simulink model "SC_Cell_Balancing"  (R2020b)
settings: Solver=VariableStepAuto  StartTime=0.0  StopTime=3000  RelTol=1e-3
model workspace (MAT data in the model file):
  C1 = Simulink.Parameter
  C1.Value = 360
  C1.DataType = 'auto'
  C1.Dimensions = [1 1]
  C10 = Simulink.Parameter
  C10.Value = 410
  C10.DataType = 'auto'
  C10.Dimensions = [1 1]
  C11 = Simulink.Parameter
  C11.Value = 420
  C11.DataType = 'auto'
  C11.Dimensions = [1 1]
  C12 = Simulink.Parameter
  C12.Value = 432
  C12.DataType = 'auto'
  C12.Dimensions = [1 1]
  C2 = Simulink.Parameter
  C2.Value = 365
  C2.DataType = 'auto'
  C2.Dimensions = [1 1]
  C3 = Simulink.Parameter
  C3.Value = 370
  C3.DataType = 'auto'
  C3.Dimensions = [1 1]
  C4 = Simulink.Parameter
  C4.Value = 375
  C4.DataType = 'auto'
  C4.Dimensions = [1 1]
  C5 = Simulink.Parameter
  C5.Value = 380
  C5.DataType = 'auto'
  C5.Dimensions = [1 1]
  C6 = Simulink.Parameter
  C6.Value = 385
  C6.DataType = 'auto'
  C6.Dimensions = [1 1]
  C7 = Simulink.Parameter
  C7.Value = 390
  C7.DataType = 'auto'
  C7.Dimensions = [1 1]
  C8 = Simulink.Parameter
  C8.Value = 395
  C8.DataType = 'auto'
  C8.Dimensions = [1 1]
  C9 = Simulink.Parameter
  C9.Value = 400
  C9.DataType = 'auto'
  C9.Dimensions = [1 1]
  R_bal = 360
  Vsc = Simulink.Parameter
  Vsc.Value = 0
  Vsc.DataType = 'auto'
  Vsc.Dimensions = [1 1]
libraries: powerlib x36, electricdrivelib x12
settings Model: OrderedModelArguments=off  Creator=reigs  LastModifiedBy=reigs

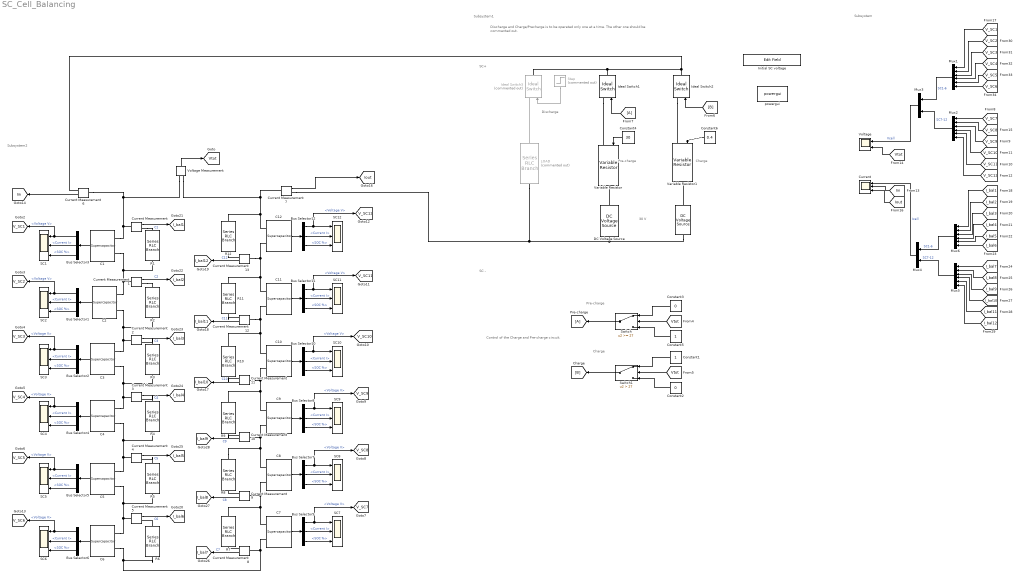
== system SC_Cell_Balancing ==
  note: Subsystem
  note: Subsystem2
  note: Subsystem1
  note: Control of the Charge and Pre-charge circuit.
  note: Charge
  note: Pre-charge
  note: SC -
  note: SC+
  note: Discharge and Charge/Precharge is to be operated only one at a time. The other one should be commented out.
  note: Discharge
  note: Pre-charge
  note: Charge
  note: 30 V
  " " : powerlib/Electrical Sources/DC Voltage Source  Amplitude=30  Measurements=None
  Bus Selector{1..12} (12 alike) : BusSelector  OutputSignals=Voltage V,Current I,SOC %
  C1 : electricdrivelib/Extra Sources/Supercapacitor  C=C1  Rdc=3.2e-3  Voltage=2.7  Ns=1  Np=1  Vinit=Vsc  Temp=25  PresetModel=off  EstParam=off  Nc=1  r=1e-9  epsilon=6.0208e-10  Ich=10  Vstern="[0.161  2.7  7.8]"  Self_dis=on  Ioc=10  Vself="[48  47.8  47.06  44.65]"  demandeplot=off  I="[10  20 100  500]"  Units=sec  Vmax=0  If=0  deltaV=0  alpha=0  sec=0
      settings: SourceProductBaseCode=PS
  C10 : electricdrivelib/Extra Sources/Supercapacitor  C=C10  Rdc=3.2e-3  Voltage=2.7  Ns=1  Np=1  Vinit=Vsc  Temp=25  PresetModel=off  EstParam=off  Nc=1  r=1e-9  epsilon=6.0208e-10  Ich=10  Vstern="[0.161  2.7  7.8]"  Self_dis=on  Ioc=10  Vself="[48  47.8  47.06  44.65]"  demandeplot=off  I="[10  20 100  500]"  Units=sec  Vmax=0  If=0  deltaV=0  alpha=0  sec=0
      settings: SourceProductBaseCode=PS
  C11 : electricdrivelib/Extra Sources/Supercapacitor  C=C11  Rdc=3.2e-3  Voltage=2.7  Ns=1  Np=1  Vinit=Vsc  Temp=25  PresetModel=off  EstParam=off  Nc=1  r=1e-9  epsilon=6.0208e-10  Ich=10  Vstern="[0.161  2.7  7.8]"  Self_dis=on  Ioc=10  Vself="[48  47.8  47.06  44.65]"  demandeplot=off  I="[10  20 100  500]"  Units=sec  Vmax=0  If=0  deltaV=0  alpha=0  sec=0
      settings: SourceProductBaseCode=PS
  C12 : electricdrivelib/Extra Sources/Supercapacitor  C=C12  Rdc=3.2e-3  Voltage=2.7  Ns=1  Np=1  Vinit=Vsc  Temp=25  PresetModel=off  EstParam=off  Nc=1  r=1e-9  epsilon=6.0208e-10  Ich=10  Vstern="[0.161  2.7  7.8]"  Self_dis=on  Ioc=10  Vself="[48  47.8  47.06  44.65]"  demandeplot=off  I="[10  20 100  500]"  Units=sec  Vmax=0  If=0  deltaV=0  alpha=0  sec=0
      settings: SourceProductBaseCode=PS
  C2 : electricdrivelib/Extra Sources/Supercapacitor  C=C2  Rdc=3.2e-3  Voltage=2.7  Ns=1  Np=1  Vinit=Vsc  Temp=25  PresetModel=off  EstParam=off  Nc=1  r=1e-9  epsilon=6.0208e-10  Ich=10  Vstern="[0.161  2.7  7.8]"  Self_dis=on  Ioc=10  Vself="[48  47.8  47.06  44.65]"  demandeplot=off  I="[10  20 100  500]"  Units=sec  Vmax=0  If=0  deltaV=0  alpha=0  sec=0
      settings: SourceProductBaseCode=PS
  C3 : electricdrivelib/Extra Sources/Supercapacitor  C=C3  Rdc=3.2e-3  Voltage=2.7  Ns=1  Np=1  Vinit=Vsc  Temp=25  PresetModel=off  EstParam=off  Nc=1  r=1e-9  epsilon=6.0208e-10  Ich=10  Vstern="[0.161  2.7  7.8]"  Self_dis=on  Ioc=10  Vself="[48  47.8  47.06  44.65]"  demandeplot=off  I="[10  20 100  500]"  Units=sec  Vmax=0  If=0  deltaV=0  alpha=0  sec=0
      settings: SourceProductBaseCode=PS
  C4 : electricdrivelib/Extra Sources/Supercapacitor  C=C4  Rdc=3.2e-3  Voltage=2.7  Ns=1  Np=1  Vinit=Vsc  Temp=25  PresetModel=off  EstParam=off  Nc=1  r=1e-9  epsilon=6.0208e-10  Ich=10  Vstern="[0.161  2.7  7.8]"  Self_dis=on  Ioc=10  Vself="[48  47.8  47.06  44.65]"  demandeplot=off  I="[10  20 100  500]"  Units=sec  Vmax=0  If=0  deltaV=0  alpha=0  sec=0
      settings: SourceProductBaseCode=PS
  C5 : electricdrivelib/Extra Sources/Supercapacitor  C=C5  Rdc=3.2e-3  Voltage=2.7  Ns=1  Np=1  Vinit=Vsc  Temp=25  PresetModel=off  EstParam=off  Nc=1  r=1e-9  epsilon=6.0208e-10  Ich=10  Vstern="[0.161  2.7  7.8]"  Self_dis=on  Ioc=10  Vself="[48  47.8  47.06  44.65]"  demandeplot=off  I="[10  20 100  500]"  Units=sec  Vmax=0  If=0  deltaV=0  alpha=0  sec=0
      settings: SourceProductBaseCode=PS
  C6 : electricdrivelib/Extra Sources/Supercapacitor  C=C6  Rdc=3.2e-3  Voltage=2.7  Ns=1  Np=1  Vinit=Vsc  Temp=25  PresetModel=off  EstParam=off  Nc=1  r=1e-9  epsilon=6.0208e-10  Ich=10  Vstern="[0.161  2.7  7.8]"  Self_dis=on  Ioc=10  Vself="[48  47.8  47.06  44.65]"  demandeplot=off  I="[10  20 100  500]"  Units=sec  Vmax=0  If=0  deltaV=0  alpha=0  sec=0
      settings: SourceProductBaseCode=PS
  C7 : electricdrivelib/Extra Sources/Supercapacitor  C=C7  Rdc=3.2e-3  Voltage=2.7  Ns=1  Np=1  Vinit=Vsc  Temp=25  PresetModel=off  EstParam=off  Nc=1  r=1e-9  epsilon=6.0208e-10  Ich=10  Vstern="[0.161  2.7  7.8]"  Self_dis=on  Ioc=10  Vself="[48  47.8  47.06  44.65]"  demandeplot=off  I="[10  20 100  500]"  Units=sec  Vmax=0  If=0  deltaV=0  alpha=0  sec=0
      settings: SourceProductBaseCode=PS
  C8 : electricdrivelib/Extra Sources/Supercapacitor  C=C8  Rdc=3.2e-3  Voltage=2.7  Ns=1  Np=1  Vinit=Vsc  Temp=25  PresetModel=off  EstParam=off  Nc=1  r=1e-9  epsilon=6.0208e-10  Ich=10  Vstern="[0.161  2.7  7.8]"  Self_dis=on  Ioc=10  Vself="[48  47.8  47.06  44.65]"  demandeplot=off  I="[10  20 100  500]"  Units=sec  Vmax=0  If=0  deltaV=0  alpha=0  sec=0
      settings: SourceProductBaseCode=PS
  C9 : electricdrivelib/Extra Sources/Supercapacitor  C=C9  Rdc=3.2e-3  Voltage=2.7  Ns=1  Np=1  Vinit=Vsc  Temp=25  PresetModel=off  EstParam=off  Nc=1  r=1e-9  epsilon=6.0208e-10  Ich=10  Vstern="[0.161  2.7  7.8]"  Self_dis=on  Ioc=10  Vself="[48  47.8  47.06  44.65]"  demandeplot=off  I="[10  20 100  500]"  Units=sec  Vmax=0  If=0  deltaV=0  alpha=0  sec=0
      settings: SourceProductBaseCode=PS
  Constant1 : Constant
  Constant2 : Constant  Value=0
  Constant3 : Constant  Value=0
  Constant4 : Constant  Value=30
  Constant5 : Constant
  Constant6 : Constant  Value=0.4
  Current : Scope  NumInputPorts=3
  Current Measurement{,1..13} (14 alike) : powerlib/Measurements/Current Measurement  PhasorSimulation=off  OutputType=Complex  PSBequivalent=0
  DC Voltage Source : powerlib/Electrical Sources/DC Voltage Source  Amplitude=30  Measurements=None
  Ideal Switch1 : powerlib/Power Electronics/Ideal Switch  Ron=0.00001  Lon=0  IC=0  Rs=1e5  Cs=inf  Measurements=off
  Ideal Switch2 : powerlib/Power Electronics/Ideal Switch  Ron=0.00001  Lon=0  IC=0  Rs=1e5  Cs=inf  Measurements=off
  Ideal Switch3 : powerlib/Power Electronics/Ideal Switch  Commented=on  Ron=0.00001  Lon=0  IC=0  Rs=1e5  Cs=inf  Measurements=off
  Initial SC voltage : EditField  LabelPosition=Hide  ShowInitialText=on  Alignment=Center
  LOAD : powerlib/Elements/Series RLC Branch  Commented=on  LConnTagsString=__new0  RConnTagsString=__new0  BranchType=R  Resistance=30  Inductance=1e-3  SetiL0=off  InitialCurrent=0  Capacitance=1e-5  Setx0=on  InitialVoltage=0  Measurements=None
  Mux{1..2,5..6} (4 alike) : Mux  Inputs=6
  Mux3 : Mux  Inputs=2
  Mux4 : Mux  Inputs=2
  R{1..12} (12 alike) : powerlib/Elements/Series RLC Branch  LConnTagsString=__new0  RConnTagsString=__new0  BranchType=R  Resistance=R_bal  Inductance=1e-3  SetiL0=off  InitialCurrent=0  Capacitance=54.3e-6  Setx0=on  InitialVoltage=160  Measurements=None
  SC{1..12} (12 alike) : Scope  NumInputPorts=3
  Step : Step  Commented=on  Time=200  SampleTime=0
  Switch : Switch  Threshold=27
  Switch1 : Switch  Criteria=u2 > Threshold  Threshold=27
  Variable Resistor : powerlib/Elements/Variable Resistor  Rabsmin=1e-3
      settings: SourceProductBaseCode=PS
  Variable Resistor1 : powerlib/Elements/Variable Resistor  Rabsmin=1e-3
      settings: SourceProductBaseCode=PS
  Voltage : Scope  NumInputPorts=2
  Voltage Measurement : powerlib/Measurements/Voltage Measurement  PhasorSimulation=off  OutputType=Complex  PSBequivalent=0
  powergui : powerlib/powergui  Priority=1  SimulationMode=Discrete  SampleTime=1e-2  frequency=60  Iterations=50  frequencyindice=0  Pbase=100e6  ErrMax=1e-4  UnitsV=kV  UnitsW=MW  buscounter=0  FunctionMessages=off  echomessages=off  EnableUseOfTLC=off  CurrentSourceSwitches=off  DisableSnubberDevices=off  DisableRonSwitches=off  DisableVfSwitches=off  DisplayEquations=off  AutomaticDiscreteSolvers=off  SolverType=Tustin/Backward Euler (TBE)  Interpol=off  ExternalGateDelay=off  methode=off  Ts=100  x0status=blocks  SPID=on  SwTol=0  HookPort=off  NonlinearTolerance=1e-4  nMaxIteration=100  ContinueOnMaxIteration=off  RestoreLinks=warning  ResistiveCurrentMeasurement=off  Frange=[0:2:500]  Ylog=off  Xlog=on  ShowGrid=off  save=off  variable=ZData  structure=0  ZoomFFT=off  StartTime=0.0  cycles=1  DisplayStyle=1  fundamental=60  FreqAxis=off  MaxFrequency=1000  frequencyindicesteady=1  RmsSteady=1  display=off
  tag scope: I_bal10=global, I_bal11=global, I_bal12=global, I_bal1=global, I_bal2=global, I_bal3=global, I_bal4=global, I_bal5=global, I_bal6=global, I_bal7=global, I_bal8=global, I_bal9=global, Iin=global, Iout=global, V_SC10=global, V_SC11=global, V_SC12=global, V_SC1=global, V_SC2=global, V_SC3=global, V_SC4=global, V_SC5=global, V_SC6=global, V_SC7=global, V_SC8=global, V_SC9=global, Vtot=global
  wires:
  [Vtot] -> Switch/2
  Constant5/1 -> Switch/3
  Switch1/1 -> [B]
  Switch/1 -> [A]
  Constant3/1 -> Switch/1
  Constant1/1 -> Switch1/1
  [Vtot] -> Switch1/2
  Constant2/1 -> Switch1/3
  Step/1 -> Ideal Switch3/1
  [A] -> Ideal Switch1/1
  Constant4/1 -> Variable Resistor/1
  [B] -> Ideal Switch2/1
  Constant6/1 -> Variable Resistor1/1
  Current Measurement3/1 -> [I_bal4]  "C4"
  Voltage Measurement/1 -> [Vtot]
  Current Measurement9/1 -> [I_bal8]  "C8"
  Current Measurement11/1 -> [I_bal10]  "C10"
  Bus Selector2/1 -> [V_SC3], SC3/1  "<Voltage V>"
  Current Measurement7/1 -> [Iout]
  C12/1 -> Bus Selector12/1
  Current Measurement/1 -> [I_bal1]  "C1"
  Bus Selector11/2 -> SC11/2  "<Current I>"
  Bus Selector5/3 -> SC5/3  "<SOC %>"
  Bus Selector6/2 -> SC6/2  "<Current I>"
  Bus Selector7/2 -> SC8/2  "<Current I>"
  Current Measurement6/1 -> [Iin]
  Bus Selector11/3 -> SC11/3  "<SOC %>"
  Bus Selector9/2 -> SC7/2  "<Current I>"
  C1/1 -> Bus Selector3/1
  Bus Selector6/1 -> [V_SC6], SC6/1  "<Voltage V>"
  Current Measurement4/1 -> [I_bal5]  "C5"
  C7/1 -> Bus Selector9/1
  C8/1 -> Bus Selector7/1
  Bus Selector8/2 -> SC9/2  "<Current I>"
  Bus Selector12/2 -> SC12/2  "<Current I>"
  Bus Selector3/3 -> SC1/3  "<SOC %>"
  C9/1 -> Bus Selector8/1
  Current Measurement10/1 -> [I_bal9]  "C9"
  Bus Selector8/3 -> SC9/3  "<SOC %>"
  C2/1 -> Bus Selector1/1
  Bus Selector1/1 -> [V_SC2], SC2/1  "<Voltage V>"
  Bus Selector5/2 -> SC5/2  "<Current I>"
  Bus Selector4/3 -> SC4/3  "<SOC %>"
  Current Measurement2/1 -> [I_bal3]  "C3"
  C11/1 -> Bus Selector11/1
  Bus Selector10/2 -> SC10/2  "<Current I>"
  Current Measurement12/1 -> [I_bal11]  "C11"
  C5/1 -> Bus Selector5/1
  Bus Selector7/1 -> [V_SC8], SC8/1  "<Voltage V>"
  Bus Selector11/1 -> [V_SC11], SC11/1  "<Voltage V>"
  Bus Selector10/3 -> SC10/3  "<SOC %>"
  C6/1 -> Bus Selector6/1
  Bus Selector7/3 -> SC8/3  "<SOC %>"
  Bus Selector2/2 -> SC3/2  "<Current I>"
  Bus Selector10/1 -> [V_SC10], SC10/1  "<Voltage V>"
  Current Measurement5/1 -> [I_bal6]  "C6"
  Bus Selector5/1 -> [V_SC5], SC5/1  "<Voltage V>"
  Bus Selector9/1 -> [V_SC7], SC7/1  "<Voltage V>"
  C4/1 -> Bus Selector4/1
  Current Measurement13/1 -> [I_bal12]  "C12"
  Bus Selector12/3 -> SC12/3  "<SOC %>"
  Bus Selector9/3 -> SC7/3  "<SOC %>"
  Bus Selector8/1 -> [V_SC9], SC9/1  "<Voltage V>"
  Bus Selector4/2 -> SC4/2  "<Current I>"
  Current Measurement1/1 -> [I_bal2]  "C2"
  Bus Selector1/2 -> SC2/2  "<Current I>"
  Bus Selector6/3 -> SC6/3  "<SOC %>"
  Current Measurement8/1 -> [I_bal7]  "C7"
  Bus Selector1/3 -> SC2/3  "<SOC %>"
  Bus Selector3/2 -> SC1/2  "<Current I>"
  Bus Selector4/1 -> [V_SC4], SC4/1  "<Voltage V>"
  C10/1 -> Bus Selector10/1
  C3/1 -> Bus Selector2/1
  Bus Selector2/3 -> SC3/3  "<SOC %>"
  Bus Selector12/1 -> [V_SC12], SC12/1  "<Voltage V>"
  Bus Selector3/1 -> [V_SC1], SC1/1  "<Voltage V>"
  [I_bal5] -> Mux6/5
  [I_bal12] -> Mux5/6
  [I_bal7] -> Mux5/1
  [I_bal8] -> Mux5/2
  [V_SC6] -> Mux1/6
  [I_bal10] -> Mux5/4
  [V_SC11] -> Mux2/5
  [Iin] -> Current/2
  [Iout] -> Current/3
  Mux3/1 -> Voltage/1  "Vcell"
  [V_SC9] -> Mux2/3
  Mux5/1 -> Mux4/2  "SC7-12"
  [V_SC8] -> Mux2/2
  [V_SC1] -> Mux1/1
  [V_SC7] -> Mux2/1
  [V_SC2] -> Mux1/2
  [I_bal9] -> Mux5/3
  Mux2/1 -> Mux3/2  "SC7-12"
  [V_SC3] -> Mux1/3
  [V_SC10] -> Mux2/4
  [V_SC4] -> Mux1/4
  [V_SC5] -> Mux1/5
  Mux6/1 -> Mux4/1  "SC1-6"
  Mux1/1 -> Mux3/1  "SC1-6"
  [I_bal11] -> Mux5/5
  [I_bal1] -> Mux6/1
  [Vtot] -> Voltage/2
  [I_bal4] -> Mux6/4
  [I_bal3] -> Mux6/3
  [I_bal2] -> Mux6/2
  [V_SC12] -> Mux2/6
  [I_bal6] -> Mux6/6
  Mux4/1 -> Current/1  "Icell"
  connections:
  Ideal Switch2/LConn1 -- Variable Resistor1/LConn1
  LOAD/LConn1 -- Ideal Switch3/LConn1
  " "/RConn1 -- Variable Resistor1/RConn1
  " "/LConn1 -- Current Measurement7/RConn1 -- LOAD/RConn1 -- DC Voltage Source/LConn1
  DC Voltage Source/RConn1 -- Variable Resistor/RConn1
  Ideal Switch1/LConn1 -- Variable Resistor/LConn1
  Ideal Switch2/RConn1 -- Current Measurement6/RConn1 -- Ideal Switch1/RConn1 -- Ideal Switch3/RConn1
  C9/LConn2 -- Current Measurement11/LConn1 -- C10/LConn1 -- R9/RConn1
  C11/LConn1 -- R10/RConn1 -- C10/LConn2 -- Current Measurement12/LConn1
  R10/LConn1 -- Current Measurement11/RConn1
  R3/LConn1 -- Current Measurement2/RConn1
  R12/LConn1 -- Current Measurement13/RConn1
  R11/LConn1 -- Current Measurement12/RConn1
  C7/LConn1 -- Current Measurement8/LConn1 -- R6/RConn1 -- C6/LConn2
  Current Measurement1/RConn1 -- R2/LConn1
  Current Measurement/RConn1 -- R1/LConn1
  R5/LConn1 -- Current Measurement4/RConn1
  Current Measurement9/RConn1 -- R8/LConn1
  Voltage Measurement/LConn1 -- Current Measurement6/LConn1 -- C1/LConn1 -- Current Measurement/LConn1
  R6/LConn1 -- Current Measurement5/RConn1
  C2/LConn2 -- C3/LConn1 -- Current Measurement2/LConn1 -- R2/RConn1
  R8/RConn1 -- Current Measurement10/LConn1 -- C9/LConn1 -- C8/LConn2
  C6/LConn1 -- Current Measurement5/LConn1 -- R5/RConn1 -- C5/LConn2
  R12/RConn1 -- Current Measurement7/LConn1 -- Voltage Measurement/LConn2 -- C12/LConn2
  Current Measurement8/RConn1 -- R7/LConn1
  R9/LConn1 -- Current Measurement10/RConn1
  R4/LConn1 -- Current Measurement3/RConn1
  C1/LConn2 -- C2/LConn1 -- Current Measurement1/LConn1 -- R1/RConn1
  C11/LConn2 -- C12/LConn1 -- Current Measurement13/LConn1 -- R11/RConn1
  C3/LConn2 -- C4/LConn1 -- Current Measurement3/LConn1 -- R3/RConn1
  C5/LConn1 -- Current Measurement4/LConn1 -- C4/LConn2 -- R4/RConn1
  Current Measurement9/LConn1 -- C7/LConn2 -- R7/RConn1 -- C8/LConn1
